simulink model "modeo_OPC_UA"  (R2024b)
settings: Solver=VariableStepAuto  StartTime=0.0  StopTime=inf  RelTol=1e-3
libraries: opcualib x2
settings Model: Creator=Usuario  LastModifiedBy=Usuario

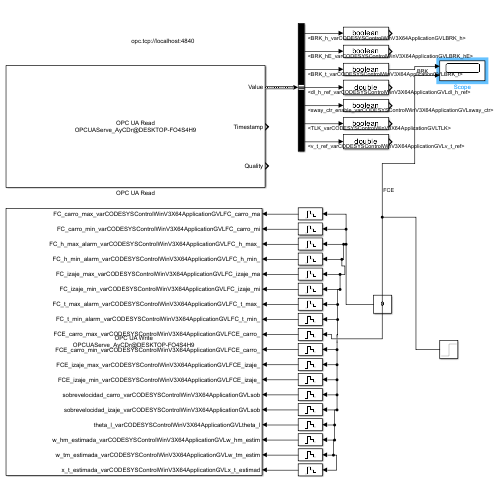
[thumbnail: Simulink's stored preview of the top-level diagram]
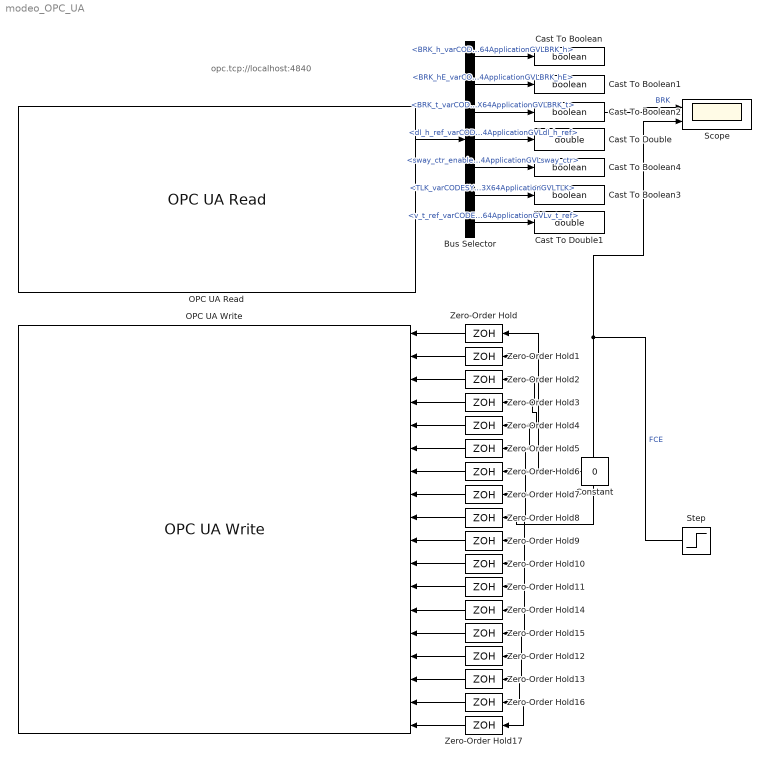
== system modeo_OPC_UA ==
  note: opc.tcp://localhost:4840
  Bus Selector : BusSelector  OutputSignals=BRK_h_varCODESYSControlWinV3X64ApplicationGVLBRK_h,BRK_hE_varCODESYSControlWinV3X64ApplicationGVLBRK_hE,BRK_t_varCODESYSControlWinV3X64ApplicationGVLBRK_t,dl_h_ref_varCODESYSControlWinV3X64ApplicationGVLdl_h_ref,sway_ctr_enable_varCODESYSControlWinV3X64ApplicationGVLsway_ctr,TLK_varCODESYSControlWinV3X64ApplicationGVLTLK,v_t_ref_varCODESYSControlWinV3X64ApplicationGVLv_t_ref
  Cast To Boolean{,1..4} (5 alike) : DataTypeConversion  OutDataTypeStr=boolean  SaturateOnIntegerOverflow=off  RndMeth=Floor
  Cast To Double : DataTypeConversion  OutDataTypeStr=double  SaturateOnIntegerOverflow=off  RndMeth=Floor
  Cast To Double1 : DataTypeConversion  OutDataTypeStr=double  SaturateOnIntegerOverflow=off  RndMeth=Floor
  Constant : Constant  Value=0
  OPC UA Read : opcualib/OPC UA Read  SelectedServer=OPCUAServe_AyCDr@DESKTOP-FO4S4H9  ServerList=OPCUAServe_AyCDr@DESKTOP-FO4S4H9  NodeList={ '1', 'BRK_h', '4', '|var|CODESYS Control Win V3 x64.Application.GVL.BRK_h', '0'; '2', 'BRK_hE', '4', '|var|CODESYS Control Win V3 x64.Application.GVL.BRK_hE', '0'; '3', 'BRK_t', '4', '|var|CODESYS Control Win V3 x64.Application.GVL.BRK_t', '0'; '4', 'dl_h_ref', '4', '|var|CODESYS Control Win V3 x64.Application.GVL.dl_h_ref', '0'; '5', 'sway_ctr_enable', '4', '|var|CODESYS Control Win V3 x64.Application.GVL.sway_ctr_enable', '0'; '6', 'TLK', '4', '|var|CODESYS Control Win V3 x64.Application.GVL.TLK', '0'; '7', 'v_t_ref', '4', '|var|CODESYS Control Win V3 x64.Application.GVL.v_t_ref', '0' }  ShowQualityPort=on  ShowTimestampPort=on  ShowTimestampPortAs=Seconds since start  SampleTime=0.020
  OPC UA Write : opcualib/OPC UA Write  SelectedServer=OPCUAServe_AyCDr@DESKTOP-FO4S4H9  ServerList=OPCUAServe_AyCDr@DESKTOP-FO4S4H9  SampleTime=0.02  NodeList={ '1', 'FC_carro_max', '4', '|var|CODESYS Control Win V3 x64.Application.GVL.FC_carro_max', '0'; '2', 'FC_carro_min', '4', '|var|CODESYS Control Win V3 x64.Application.GVL.FC_carro_min', '0'; '3', 'FC_h_max_alarm', '4', '|var|CODESYS Control Win V3 x64.Application.GVL.FC_h_max_alarm', '0'; '4', 'FC_h_min_alarm', '4', '|var|CODESYS Control Win V3 x64.Application.GVL.FC_h_min_alarm', '0'; '5', 'FC_izaje_max', '4', '|var|CODESYS Control Win V3 x64.Application.GVL.FC_izaje_max', '0'; '6', 'FC_izaje_min', '4', '|var|CODESYS Control Win V3 x64.Application.GVL.FC_izaje_min', '0'; '7', 'FC_t_max_alarm', '4', '|var|CODESYS Control Win V3 x64.Application.GVL.FC_t_max_alarm', '0'; '8', 'FC_t_min_alarm', '4', '|var|CODESYS Control Win V3 x64.Application.GVL.FC_t_min_alarm', '0'; '9', 'FCE_carro_max', '4', '|var|CODESYS Control Win V3 x64.Application.GVL.FCE_carro_max', '0'; '10', 'FCE_carro_min', '4', '|var|CODESYS Control Win V3 x64.Application.GVL.FCE_carro_min', '0'; '11', 'FCE_izaje_max', '4', '|var|CODESYS Control Win V3 x64.Application.GVL.FCE_izaje_max', '0'; '12', 'FCE_izaje_min', '4', '|var|CODESYS Control Win V3 x64.Application.GVL.FCE_izaje_min', '0'; '13', 'sobrevelocidad_carro', '4', '|var|CODESYS Control Win V3 x64.Application.GVL.sobrevelocidad_carro', '0'; '14', 'sobrevelocidad_izaje', '4', '|var|CODESYS Control Win V3 x64.Application.GVL.sobrevelocidad_izaje', '0'; '15', 'theta_l', '4', '|var|CODESYS Control Win V3 x64.Application.GVL.theta_l', '0'; '16', 'w_hm_estimada', '4', '|var|CODESYS Control Win V3 x64.Application.GVL.w_hm_estimada', '0'; '17', 'w_tm_estimada', '4', '|var|CODESYS Control Win V3 x64.Application.GVL.w_tm_estimada', '0'; '18', 'x_t_estimada', '4', '|var|CODESYS Control Win V3 x64.Application.GVL.x_t_estimada', '0' }
  Scope : Scope  NumInputPorts=2
  Step : Step  Time=20  SampleTime=0
  Zero-Order Hold{,1..17} (18 alike) : ZeroOrderHold  SampleTime=-1
  wires:
  OPC UA Read/1 -> Bus Selector/1
  Bus Selector/2 -> Cast To Boolean1/1  "<BRK_hE_varCODESYSControlWinV3X64ApplicationGVLBRK_hE>"
  Bus Selector/3 -> Cast To Boolean2/1  "<BRK_t_varCODESYSControlWinV3X64ApplicationGVLBRK_t>"
  Bus Selector/5 -> Cast To Boolean4/1  "<sway_ctr_enable_varCODESYSControlWinV3X64ApplicationGVLsway_ctr>"
  Bus Selector/6 -> Cast To Boolean3/1  "<TLK_varCODESYSControlWinV3X64ApplicationGVLTLK>"
  Bus Selector/4 -> Cast To Double/1  "<dl_h_ref_varCODESYSControlWinV3X64ApplicationGVLdl_h_ref>"
  Bus Selector/7 -> Cast To Double1/1  "<v_t_ref_varCODESYSControlWinV3X64ApplicationGVLv_t_ref>"
  Zero-Order Hold/1 -> OPC UA Write/1
  Zero-Order Hold1/1 -> OPC UA Write/2
  Zero-Order Hold2/1 -> OPC UA Write/3
  Zero-Order Hold3/1 -> OPC UA Write/4
  Zero-Order Hold4/1 -> OPC UA Write/5
  Zero-Order Hold5/1 -> OPC UA Write/6
  Zero-Order Hold6/1 -> OPC UA Write/7
  Zero-Order Hold7/1 -> OPC UA Write/8
  Zero-Order Hold8/1 -> OPC UA Write/9
  Zero-Order Hold9/1 -> OPC UA Write/10
  Zero-Order Hold10/1 -> OPC UA Write/11
  Zero-Order Hold11/1 -> OPC UA Write/12
  Zero-Order Hold14/1 -> OPC UA Write/13
  Zero-Order Hold15/1 -> OPC UA Write/14
  Zero-Order Hold12/1 -> OPC UA Write/15
  Zero-Order Hold13/1 -> OPC UA Write/16
  Zero-Order Hold16/1 -> OPC UA Write/17
  Zero-Order Hold17/1 -> OPC UA Write/18
  Constant/1 -> Zero-Order Hold/1, Zero-Order Hold1/1, Zero-Order Hold4/1, Zero-Order Hold17/1, Zero-Order Hold16/1, Zero-Order Hold13/1, Zero-Order Hold12/1, Zero-Order Hold15/1, Zero-Order Hold14/1, Zero-Order Hold11/1, Zero-Order Hold10/1, Zero-Order Hold9/1, Zero-Order Hold7/1, Zero-Order Hold6/1, Zero-Order Hold5/1, Zero-Order Hold3/1, Zero-Order Hold2/1
  Step/1 -> Zero-Order Hold8/1, Scope/2  "FCE"
  Cast To Boolean2/1 -> Scope/1  "BRK"
  Bus Selector/1 -> Cast To Boolean/1  "<BRK_h_varCODESYSControlWinV3X64ApplicationGVLBRK_h>"
